simulink model "untitled"  (Simulink 4.00)
settings: Solver=ode45  StartTime=0.0  StopTime=10.0  RelTol=1e-3
settings Model: LastModifiedBy=Хозяин

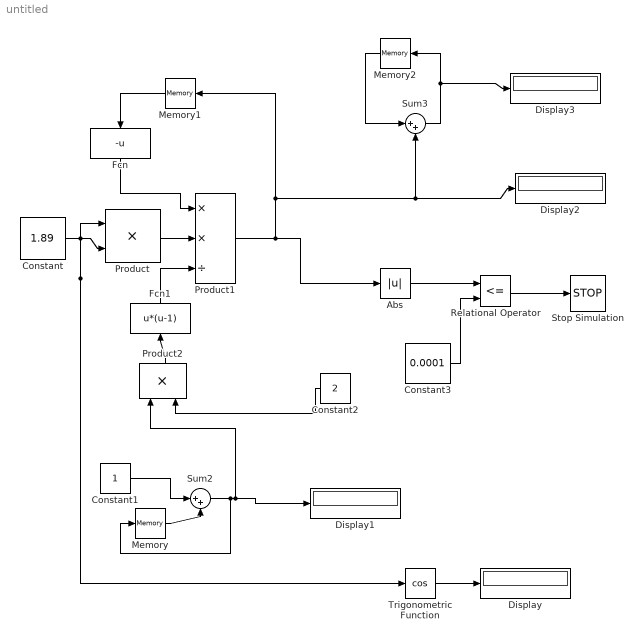
== system untitled ==
  Abs : Abs  SaturateOnIntegerOverflow=on
  Constant : Constant  Value=1.89  VectorParams1D=off
  Constant1 : Constant  Value=1
  Constant2 : Constant  Orientation=left  Value=2
  Constant3 : Constant  Value=0.0001  VectorParams1D=off
  Display{,1..3} (4 alike) : Display
      settings: Format=short
  Fcn : Fcn  Orientation=down  Expr=-u
  Fcn1 : Fcn  Orientation=up  Expr=u*(u-1)
  Memory : Memory  X0=0  InheritSampleTime=off
      settings: RTWStateStorageClass=Auto
  Memory1 : Memory  Orientation=left  X0=1  InheritSampleTime=off
      settings: RTWStateStorageClass=Auto
  Memory2 : Memory  Orientation=left  X0=1  InheritSampleTime=off
      settings: RTWStateStorageClass=Auto
  Product : Product  Inputs=2  Multiplication=Element-wise(.*)  SaturateOnIntegerOverflow=on
  Product1 : Product  Inputs=**/  Multiplication=Element-wise(.*)  SaturateOnIntegerOverflow=on
  Product2 : Product  Orientation=up  Inputs=2  Multiplication=Element-wise(.*)  SaturateOnIntegerOverflow=on
  Relational Operator : RelationalOperator  Operator=<=
  Stop Simulation : Stop
  Sum2 : Sum  Inputs=|++  SaturateOnIntegerOverflow=on
  Sum3 : Sum  Inputs=|++  SaturateOnIntegerOverflow=on
  Trigonometric Function : Trigonometry  Operator=cos  OutputSignalType=auto
  wires:
  Constant/1 -> Product/1, Product/2, Trigonometric Function/1
  Trigonometric Function/1 -> Display/1
  Product/1 -> Product1/2
  Constant1/1 -> Sum2/1
  Sum2/1 -> Memory/1, Display1/1, Product2/1
  Product1/1 -> Abs/1, Memory1/1, Display2/1, Sum3/2
  Abs/1 -> Relational Operator/1
  Constant3/1 -> Relational Operator/2
  Relational Operator/1 -> Stop Simulation/1
  Fcn/1 -> Product1/1
  Sum3/1 -> Memory2/1, Display3/1
  Memory2/1 -> Sum3/1
  Memory1/1 -> Fcn/1
  Constant2/1 -> Product2/2
  Memory/1 -> Sum2/2
  Product2/1 -> Fcn1/1
  Fcn1/1 -> Product1/3
